simulink model "example2"  (R2015b)
settings: Solver=VariableStepAuto  StartTime=0.0  StopTime=100  RelTol=1e-3
undefined symbols (not defined in the file): A, B, C, D
settings Model: Creator=pk  LastModifiedBy=pk

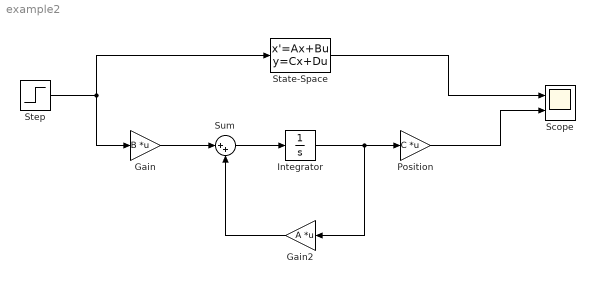
== system example2 ==
  Gain : Gain  Gain=B  Multiplication=Matrix(K*u)
  Gain2 : Gain  Gain=A  Multiplication=Matrix(K*u)
  Integrator : Integrator
  Position : Gain  Gain=C  Multiplication=Matrix(K*u)
  Scope : Scope  NumInputPorts=2
  State-Space : StateSpace  A=A  B=B  C=C  D=D  X0=0
  Step : Step  SampleTime=0
  Sum : Sum  Inputs=|++
  wires:
  Step/1 -> State-Space/1, Gain/1
  Gain/1 -> Sum/1
  Sum/1 -> Integrator/1
  Integrator/1 -> Gain2/1, Position/1
  Gain2/1 -> Sum/2
  Position/1 -> Scope/2
  State-Space/1 -> Scope/1
